simulink model "chap6_1sim"  (Simulink 7.7)
settings: Solver=ode45  StartTime=0.0  StopTime=10  RelTol=1e-3
settings Model: Creator=ljk  LastModifiedBy=ljk  ExtModeTrigMode=oneshot  ExtModeArmWhenConnect=off
settings DataIOCC: LimitDataPoints=off  SignalLoggingName=sigsOut
settings OptimizationCC: BooleanDataType=off
settings DebuggingCC: SaveWithParameterizedLinksMsg=none  SignalResolutionControl=TryResolveAllWithWarning  SolverPrmCheckMsg=none  MultiTaskDSMMsg=warning  MultiTaskCondExecSysMsg=none  StrictBusMsg=None
settings HardwareCC: TargetUnknown=on
settings RTWCC: IncludeERTFirstTime=on

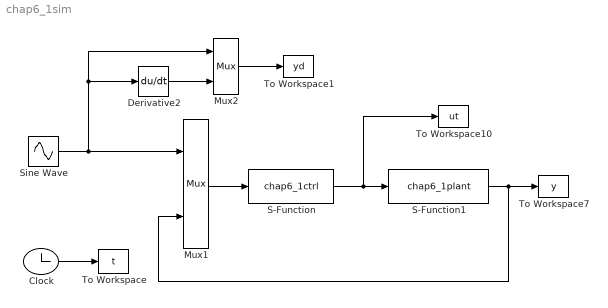
== system chap6_1sim ==
  Clock : Clock
  Derivative2 : Derivative
  Mux1 : Mux  Inputs=2
  Mux2 : Mux  Inputs=2
  S-Function : S-Function  FunctionName=chap6_1ctrl  EnableBusSupport=off
  S-Function1 : S-Function  FunctionName=chap6_1plant  EnableBusSupport=off
  Sine Wave : Sin  Amplitude=0.10  Frequency=pi  SampleTime=0
  To Workspace : ToWorkspace  VariableName=t  SampleTime=-1  SaveFormat=Array
  To Workspace1 : ToWorkspace  VariableName=yd  SampleTime=-1  SaveFormat=Array
  To Workspace10 : ToWorkspace  VariableName=ut  SampleTime=-1  SaveFormat=Array
  To Workspace7 : ToWorkspace  VariableName=y  SampleTime=-1  SaveFormat=Array
  wires:
  Mux1/1 -> S-Function/1
  S-Function/1 -> S-Function1/1, To Workspace10/1
  S-Function1/1 -> Mux1/2, To Workspace7/1
  Sine Wave/1 -> Derivative2/1, Mux2/1, Mux1/1
  Clock/1 -> To Workspace/1
  Mux2/1 -> To Workspace1/1
  Derivative2/1 -> Mux2/2
